simulink model "control_simulink"  (R2017b)
settings: Solver=VariableStepAuto  StartTime=0.0  StopTime=10.0  RelTol=1e-3
values from neighbouring files (symbols this model uses):
  D = coefD    [coefficent.m]
  N = coufN    [coefficent.m]
libraries: simulink x2
settings Model: Creator=Ahmad Mustafa  LastModifiedBy=Ahmad Mustafa
settings DataIOCC: ExternalInput=[N, D, M]

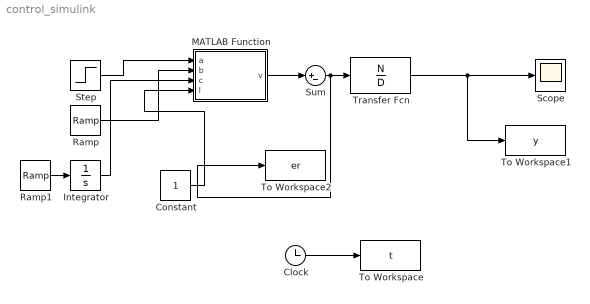
== system control_simulink ==
  Clock : Clock
  Constant : Constant
  Integrator : Integrator
  MATLAB Function : MATLAB Function  TreatAsAtomicUnit=on
  Ramp : simulink/Sources/Ramp  slope=1  start=0  X0=0
  Ramp1 : simulink/Sources/Ramp  slope=1  start=0  X0=0
  Scope : Scope
  Step : Step  Time=0  SampleTime=0
  Sum : Sum  Inputs=|+-
  To Workspace : ToWorkspace  VariableName=t  SampleTime=-1
  To Workspace1 : ToWorkspace  VariableName=y  SampleTime=-1
  To Workspace2 : ToWorkspace  VariableName=er  SampleTime=-1
  Transfer Fcn : TransferFcn  Numerator=N  Denominator=D
  wires:
  Transfer Fcn/1 -> To Workspace1/1, Scope/1
  MATLAB Function/1(v) -> Sum/1
  Ramp1/1 -> Integrator/1
  Ramp/1 -> MATLAB Function/2(b)
  Step/1 -> MATLAB Function/1(a)
  Integrator/1 -> MATLAB Function/3(c)
  Constant/1 -> MATLAB Function/4(l)
  Clock/1 -> To Workspace/1
  Sum/1 -> To Workspace2/1, Transfer Fcn/1

== matlab function control_simulink/MATLAB Function ==
  data: a input; v output; b input; c input; l input
function v = fcn(a , b ,c,l)
if l == 1
        v=a;
elseif l == 2 
        v=b;
else
        v=c;
end
